simulink model "fp_arith_1"  (Simulink 7.6)
settings: Solver=ode45  StartTime=0.0  StopTime=1  RelTol=1e-3
settings Model: Creator=jordan  LastModifiedBy=jordan

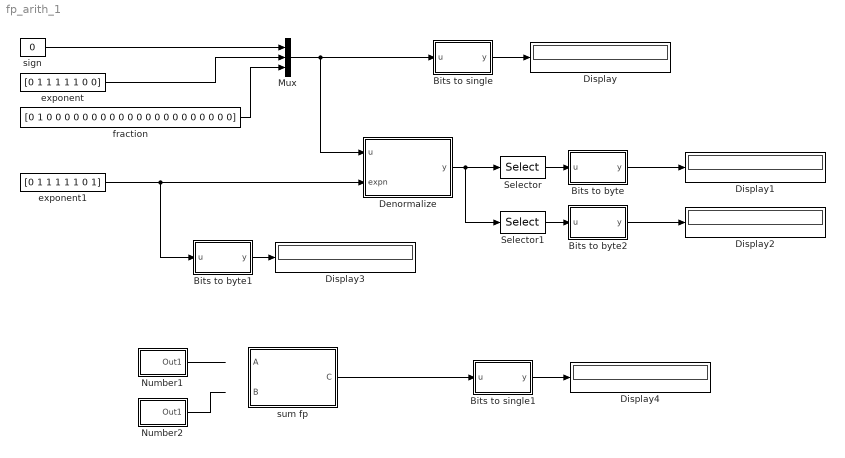
== system fp_arith_1 ==
  Bits to byte : Stateflow chart  TreatAsAtomicUnit=on
  Bits to byte1 : Stateflow chart  TreatAsAtomicUnit=on
  Bits to byte2 : Stateflow chart  TreatAsAtomicUnit=on
  Bits to single : Stateflow chart  TreatAsAtomicUnit=on
  Bits to single1 : Stateflow chart  TreatAsAtomicUnit=on
  Denormalize : Stateflow chart  TreatAsAtomicUnit=on
  Display{,1..4} (5 alike) : Display
  Mux : Mux  Inputs=3
  Number1 : Subsystem
  Number2 : Subsystem
  Selector : Selector  InputPortWidth=33  IndexOptions=Index vector (dialog)  Indices=[2:9]  OutputSizes=1
  Selector1 : Selector  InputPortWidth=33  IndexOptions=Index vector (dialog)  Indices=[10:33]  OutputSizes=1
  exponent : Constant  Value=[0 1 1 1 1 1 0 0]  OutDataTypeStr=boolean
  exponent1 : Constant  Value=[0 1 1 1 1 1 0 1]  OutDataTypeStr=boolean
  fraction : Constant  Value=[0 1 0 0 0 0 0 0 0 0 0 0 0 0 0 0 0 0 0 0 0 0 0]  OutDataTypeStr=boolean
  sign : Constant  Value=0  OutDataTypeStr=boolean
  sum fp : Stateflow chart  TreatAsAtomicUnit=on
  wires:
  sign/1 -> Mux/1
  exponent/1 -> Mux/2
  fraction/1 -> Mux/3
  Mux/1 -> Bits to single/1(u), Denormalize/1(u)
  Bits to single/1(y) -> Display/1
  exponent1/1 -> Denormalize/2(expn), Bits to byte1/1(u)
  Denormalize/1(y) -> Selector/1, Selector1/1
  Selector/1 -> Bits to byte/1(u)
  Selector1/1 -> Bits to byte2/1(u)
  Bits to byte/1(y) -> Display1/1
  Bits to byte1/1(y) -> Display3/1
  Bits to byte2/1(y) -> Display2/1
  Number1/1(Out1) -> ?
  Number2/1(Out1) -> ?
  Bits to single1/1(y) -> Display4/1
  sum fp/1(C) -> Bits to single1/1(u)

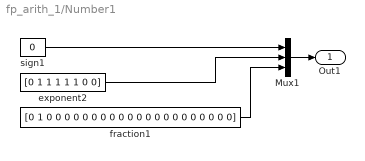
== system fp_arith_1/Number1 ==
  Mux1 : Mux  Inputs=3
  exponent2 : Constant  Value=[0 1 1 1 1 1 0 0]  OutDataTypeStr=boolean
  fraction1 : Constant  Value=[0 1 0 0 0 0 0 0 0 0 0 0 0 0 0 0 0 0 0 0 0 0 0]  OutDataTypeStr=boolean
  sign1 : Constant  Value=0  OutDataTypeStr=boolean
  Out1 : Outport
  wires:
  sign1/1 -> Mux1/1
  exponent2/1 -> Mux1/2
  fraction1/1 -> Mux1/3
  Mux1/1 -> Out1/1

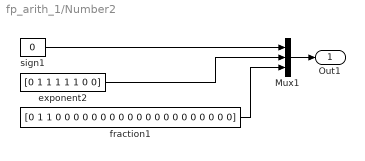
== system fp_arith_1/Number2 ==
  Mux1 : Mux  Inputs=3
  exponent2 : Constant  Value=[0 1 1 1 1 1 0 0]  OutDataTypeStr=boolean
  fraction1 : Constant  Value=[0 1 1 0 0 0 0 0 0 0 0 0 0 0 0 0 0 0 0 0 0 0 0]  OutDataTypeStr=boolean
  sign1 : Constant  Value=0  OutDataTypeStr=boolean
  Out1 : Outport
  wires:
  Mux1/1 -> Out1/1
  fraction1/1 -> Mux1/3
  exponent2/1 -> Mux1/2
  sign1/1 -> Mux1/1

== matlab function Denormalize ==
  data: u input boolean; y output boolean size=33; expn input double; bufy parameter boolean size=33
function y = fcn(u,expn, bufy)
%#eml

%bufy=uint8(zeros(1,33));
bufy(1)=u(1);
e1=uint8(0); e2=uint8(0);
u1=uint8(u); u2=uint8(expn);
for ind=1:8
    e1=e1+bitshift(u1(ind+1),8-ind);
    e2=e2+bitshift(u2(ind),8-ind);
end
frac=[1 u(10:32)'];
%e2 is always bigger than e1
buf=e2-e1;
frac_old=frac;
if (buf>0)
    frac(1:buf)=0;
    frac(buf+1:end)=frac_old(1:end-buf);
end
bufy(2:9)=expn;
bufy(10:33)=frac;
y=bufy;

== matlab function Bits to single ==
  data: u input boolean; y output single
function y = fcn(u)
%#eml

u1=uint32(u);
buf=uint32(0);
for ind=1:32
    buf=buf+bitshift(u1(ind),32-ind);
end
y = typecast(buf,'single');

== matlab function Bits to byte ==
  data: u input boolean; y output uint8
function y = fcn(u)
%#eml

u1=uint8(u);
buf=uint8(0);
for ind=1:8
    buf=buf+bitshift(u1(ind),8-ind);
end
y = typecast(buf,'uint8');

== matlab function Bits to byte1 ==
  data: u input boolean; y output uint8
function y = fcn(u)
%#eml

u1=uint8(u);
buf=uint8(0);
for ind=1:8
    buf=buf+bitshift(u1(ind),8-ind);
end
y = typecast(buf,'uint8');

== matlab function Bits to byte2 ==
  data: u input boolean; y output uint32
function y = fcn(u)
%#eml

u1=uint32(u);
buf=uint32(0);
for ind=1:24
    buf=buf+bitshift(u1(ind),24-ind);
end
y = buf;

== matlab function sum fp ==
  data: A input boolean size=32; C output boolean size=33; B input boolean size=32; bufy parameter boolean size=33
function C = fcn(A,B, bufy)
%#eml

e1=uint8(0); e2=uint8(0);
u1=uint8(A); u2=uint8(B);
for ind=1:8
    e1=e1+bitshift(u1(ind+1),8-ind);
    e2=e2+bitshift(u2(ind+1),8-ind);
end
%e2 is always bigger than e1
exch=0;
if e1>e2
    c=e2;
    e2=e1;
    e1=c;
    frac1=[1 B(10:32)'];
    frac2=[1 A(10:32)'];
    exch=1;
else
    frac1=[1 A(10:32)'];
    frac2=[1 B(10:32)'];
end

%denormalize frac1, to have the same exponent as frac2
if (e1<e2)
    buf=e2-e1;
    frac_old=frac1;
    if (buf>0)
        frac1(1:buf)=0;
        frac1(buf+1:end)=frac_old(1:end-buf);
    end
end

%find if the two numbers are with the same sign
sn=bitxor(u1(1),u2(1));
if ~sn
    bufy(1)=A(1);
    frac=frac1;
    c1=uint8(0);
    for ind=0:23
        x=uint8(frac1(24-ind));
        y=uint8(frac2(24-ind));
        frac(24-ind)=bitor(bitand(~c1,bitxor(x,y)),bitand(c1,bitor(bitand(~x,~y),bitand(x,y))));
        c1=x&y|(c1&bitxor(x,y));
    end
else
end

%normalize result
buf=uint8(0);
for ind=1:24
    if (frac(ind))
        break;
    else
        buf=buf+1;
    end
end
frac_old=frac;
frac=0;
if (buf>0)
    frac(1:24-buf)=frac_old(buf:end);
end
e2=e2-buf;
for ind=0:7
    bufy(2:9)=bitand(e2,2^(8-ind));
end
bufy(10:32)=frac(2:33);
C=bufy;

== matlab function Bits to single1 ==
  data: u input boolean; y output single
function y = fcn(u)
%#eml

u1=uint32(u);
buf=uint32(0);
for ind=1:32
    buf=buf+bitshift(u1(ind),32-ind);
end
y = typecast(buf,'single');
